simulink model "BLDC_120degree_speed_control"  (R2022b)
settings: Solver=VariableStepAuto  StartTime=0.0  StopTime=0.5  FixedStep=0.000001  MinStep=0.000001  RelTol=1e-3
values from neighbouring files (symbols this model uses):
  B = 0.0005    [bldc_params.m]
  J = 0.0002    [bldc_params.m]
  Lamda_p = Kb * pole/2    (= 0.1046)    [bldc_params.m]
  Ls_Lm = 5.21e-3    (= 0.00521)    [bldc_params.m]
  pole = 4    [bldc_params.m]
  Rs = 0.7    [bldc_params.m]
  T_rate = 1.78    [bldc_params.m]
libraries: slpidlib x1, spsTriangleGeneratorLib x1
settings Model: Creator=jack  LastModifiedBy=jack

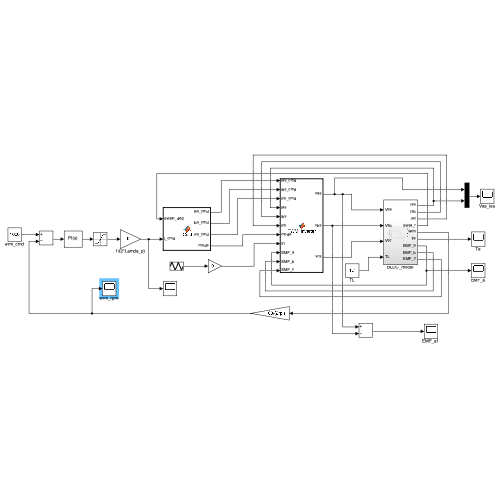
[thumbnail: Simulink's stored preview of the top-level diagram]
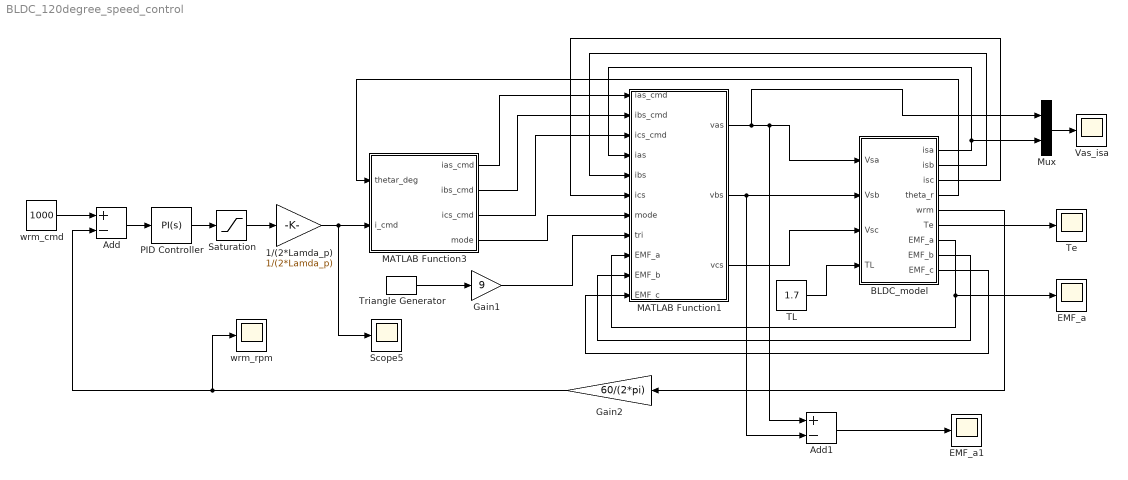
== system BLDC_120degree_speed_control ==
  1/(2*Lamda_p) : Gain  Gain=1/(2*Lamda_p)
  Add : Sum  Inputs=+-
  Add1 : Sum  Inputs=+-
  BLDC_model : Subsystem
  EMF_a : Scope
  EMF_a1 : Scope
  Gain1 : Gain  Gain=9
  Gain2 : Gain  Gain=60/(2*pi)
  MATLAB Function1 : MATLAB Function  TreatAsAtomicUnit=on
  MATLAB Function3 : MATLAB Function  TreatAsAtomicUnit=on
  Mux : Mux  Inputs=2
  PID Controller : slpidlib/PID Controller  Controller=PI  Form=Parallel  TimeDomain=Continuous-time  UseExternalTs=off  SampleTime=-1  IntegratorMethod=Forward Euler  FilterMethod=Forward Euler  ControllerParametersSource=internal  P=0.03  I=0.25  UseKiTs=off  D=0  N=100  UseFilter=on  TunerSelectOption=Transfer Function Based (PID Tuner App)  InitialConditionSource=internal  InitialConditionForIntegrator=0  InitialConditionForFilter=0  DifferentiatorICPrevScaledInput=0  ExternalReset=none  TrackingMode=off  Kt=1  LimitOutput=off  SatLimitsSource=internal  UpperSaturationLimit=inf  LowerSaturationLimit=-inf  LinearizeAsGain=on  AntiWindupMode=none  Kb=1  LimitIntegrator=off  UpperIntegratorSaturationLimit=inf  LowerIntegratorSaturationLimit=-inf  POutMin=[]  POutMax=[]  IOutMin=[]  IOutMax=[]  DOutMin=[]  DOutMax=[]  NOutMin=[]  NOutMax=[]  SumOutMin=[]  SumOutMax=[]  SaturationOutMin=[]  SaturationOutMax=[]  PParamMin=[]  PParamMax=[]  IParamMin=[]  IParamMax=[]  DParamMin=[]  DParamMax=[]  NParamMin=[]  NParamMax=[]  KbParamMin=[]  KbParamMax=[]  KtParamMin=[]  KtParamMax=[]  KbOutMin=[]  KbOutMax=[]  KtOutMin=[]  KtOutMax=[]  IntegratorOutMin=[]  IntegratorOutMax=[]  FilterOutMin=[]  FilterOutMax=[]  SumI1OutMin=[]  SumI1OutMax=[]  SumI2OutMin=[]  SumI2OutMax=[]  SumI3OutMin=[]  SumI3OutMax=[]  SumI4OutMin=[]  SumI4OutMax=[]  SumDOutMin=[]  SumDOutMax=[]  DifferentiatorOutMin=[]  DifferentiatorOutMax=[]  FilterDiffOutCoefMin=[]  FilterDiffOutCoefMax=[]  ReciprocalOutMin=[]  ReciprocalOutMax=[]  SumDenOutMin=[]  SumDenOutMax=[]  SumNumOutMin=[]  SumNumOutMax=[]  DivideOutMin=[]  DivideOutMax=[]  UdiffTsProdOutMin=[]  UdiffTsProdOutMax=[]  NTsProdOutMin=[]  NTsProdOutMax=[]  UintegralTsProdOutMin=[]  UintegralTsProdOutMax=[]  UngainTsProdOutMin=[]  UngainTsProdOutMax=[]  ClampingZeroOutDataTypeStr=Inherit: Inherit via back propagation  ClampingZeroOutMin=[]  ClampingZeroOutMax=[]  FilterDenConstantOutDataTypeStr=Inherit: Inherit via back propagation  FilterDenConstantOutMin=[]  FilterDenConstantOutMax=[]  PCopyOutDataTypeStr=Inherit: Inherit via back propagation  PCopyOutMin=[]  PCopyOutMax=[]  NCopyOutDataTypeStr=Inherit: Inherit via back propagation  NCopyOutMin=[]  NCopyOutMax=[]  IntegratorContinuousStateAttributes=''  IntegratorStateMustResolveToSignalObject=off  IntegratorRTWStateStorageClass=Auto  FilterContinuousStateAttributes=''  FilterStateMustResolveToSignalObject=off  FilterRTWStateStorageClass=Auto  ParallelPVariant=InternalParameters  IdealPVariant=Disabled  IVariant=InternalParameters  DVariant=Disabled  IntegratorVariant=Continuous  SatVariant=Disabled  AWVariant=Passthrough  PCopyVariant=Disabled  TRVariant=Disabled  FdbkBlocksVariant=Forward  IdealPFdbkVariant=Disabled  SatFdbkVariant=Disabled  DerivativeFilterVariant=Disabled  NVariant=Disabled  NCopyVariant=Disabled_SignalSpec  FilterICVariant=Disabled  IntegratorICVariant=InternalICs  ExternalResetVariant=Disabled  TRSumVariant=Passthrough  SumFdbkVariant=Disabled  SumVariant=Sum_PI  TsampFilterVariant=InternalTs  TsampNgainVariant=Passthrough  TsampIntegralVariant=Passthrough  ExternalSaturationOutDataTypeStr=Inherit: Same as second input
  Saturation : Saturate  UpperLimit=2*T_rate  LowerLimit=-2*T_rate
  Scope5 : Scope
  TL : Constant  Value=1.7
  Te : Scope
  Triangle Generator : spsTriangleGeneratorLib/Triangle Generator  Freq=4000  Phase=90  Ts=0
  Vas_isa : Scope
  wrm_cmd : Constant  Value=1000
  wrm_rpm : Scope
  wires:
  wrm_cmd/1 -> Add/1
  Add/1 -> PID Controller/1
  PID Controller/1 -> Saturation/1
  BLDC_model/5(wrm) -> Gain2/1
  1/(2*Lamda_p)/1 -> MATLAB Function3/2(i_cmd), Scope5/1
  MATLAB Function3/1(ias_cmd) -> MATLAB Function1/1(ias_cmd)
  MATLAB Function3/2(ibs_cmd) -> MATLAB Function1/2(ibs_cmd)
  MATLAB Function3/3(ics_cmd) -> MATLAB Function1/3(ics_cmd)
  MATLAB Function3/4(mode) -> MATLAB Function1/7(mode)
  BLDC_model/2(isb) -> MATLAB Function1/5(ibs)
  BLDC_model/3(isc) -> MATLAB Function1/6(ics)
  Triangle Generator/1 -> Gain1/1
  Gain1/1 -> MATLAB Function1/8(tri)
  MATLAB Function1/1(vas) -> Mux/1, Add1/1, BLDC_model/1(Vsa)
  MATLAB Function1/2(vbs) -> Add1/2, BLDC_model/2(Vsb)
  MATLAB Function1/3(vcs) -> BLDC_model/3(Vsc)
  TL/1 -> BLDC_model/4(TL)
  BLDC_model/4(theta_r) -> MATLAB Function3/1(thetar_deg)
  Gain2/1 -> wrm_rpm/1, Add/2
  BLDC_model/1(isa) -> MATLAB Function1/4(ias), Mux/2
  Saturation/1 -> 1/(2*Lamda_p)/1
  BLDC_model/9(EMF_c) -> MATLAB Function1/11(EMF_c)
  BLDC_model/8(EMF_b) -> MATLAB Function1/10(EMF_b)
  BLDC_model/7(EMF_a) -> EMF_a/1, MATLAB Function1/9(EMF_a)
  Mux/1 -> Vas_isa/1
  Add1/1 -> EMF_a1/1
  BLDC_model/6(Te) -> Te/1

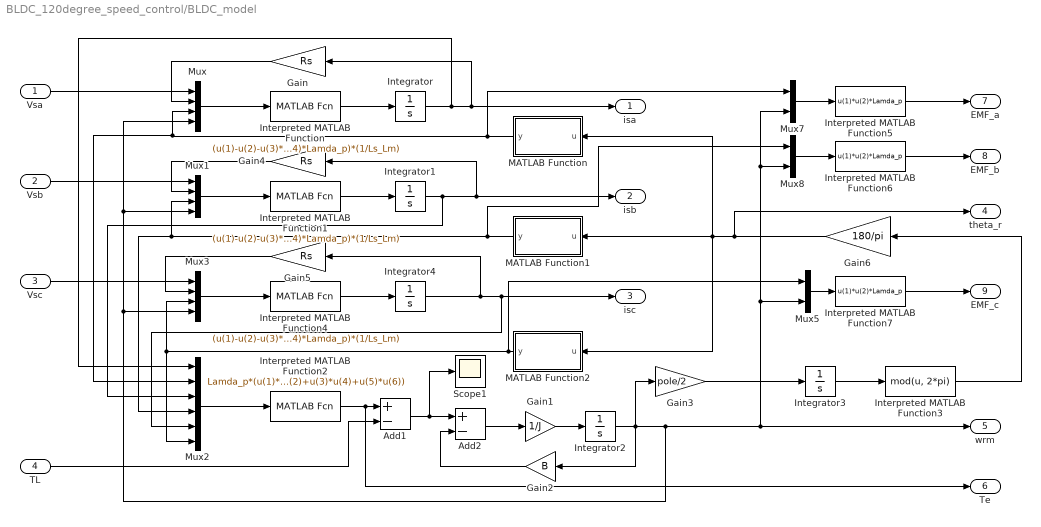
== system BLDC_120degree_speed_control/BLDC_model ==
  Vsa : Inport
  Vsb : Inport  Port=2
  Vsc : Inport  Port=3
  TL : Inport  Port=4
  Add1 : Sum  Inputs=+-
  Add2 : Sum  Inputs=+-
  Gain : Gain  Gain=Rs
  Gain1 : Gain  Gain=1/J
  Gain2 : Gain  Gain=B
  Gain3 : Gain  Gain=pole/2
  Gain4 : Gain  Gain=Rs
  Gain5 : Gain  Gain=Rs
  Gain6 : Gain  Gain=180/pi
  Integrator{,1..4} (5 alike) : Integrator
  Interpreted MATLAB Function : MATLABFcn  MATLABFcn=(u(1)-u(2)-u(3)*u(4)*Lamda_p)*(1/Ls_Lm)
  Interpreted MATLAB Function1 : MATLABFcn  MATLABFcn=(u(1)-u(2)-u(3)*u(4)*Lamda_p)*(1/Ls_Lm)
  Interpreted MATLAB Function2 : MATLABFcn  MATLABFcn=Lamda_p*(u(1)*u(2)+u(3)*u(4)+u(5)*u(6))
  Interpreted MATLAB Function3 : MATLABFcn  MATLABFcn=mod(u, 2*pi)
  Interpreted MATLAB Function4 : MATLABFcn  MATLABFcn=(u(1)-u(2)-u(3)*u(4)*Lamda_p)*(1/Ls_Lm)
  Interpreted MATLAB Function5 : MATLABFcn  MATLABFcn=u(1)*u(2)*Lamda_p
  Interpreted MATLAB Function6 : MATLABFcn  MATLABFcn=u(1)*u(2)*Lamda_p
  Interpreted MATLAB Function7 : MATLABFcn  MATLABFcn=u(1)*u(2)*Lamda_p
  MATLAB Function : MATLAB Function  TreatAsAtomicUnit=on
  MATLAB Function1 : MATLAB Function  TreatAsAtomicUnit=on
  MATLAB Function2 : MATLAB Function  TreatAsAtomicUnit=on
  Mux : Mux
  Mux1 : Mux
  Mux2 : Mux  Inputs=6
  Mux3 : Mux
  Mux5 : Mux  Inputs=2
  Mux7 : Mux  Inputs=2
  Mux8 : Mux  Inputs=2
  Scope1 : Scope
  isa : Outport
  isb : Outport  Port=2
  isc : Outport  Port=3
  theta_r : Outport  Port=4
  wrm : Outport  Port=5
  Te : Outport  Port=6
  EMF_a : Outport  Port=7
  EMF_b : Outport  Port=8
  EMF_c : Outport  Port=9
  wires:
  Gain5/1 -> Mux3/2
  Gain2/1 -> Add2/2
  Mux1/1 -> Interpreted MATLAB Function1/1
  Integrator2/1 -> Gain3/1, Mux1/4, Mux/4, Mux3/4, wrm/1, Mux7/2, Mux8/2, Mux5/2, Gain2/1
  Interpreted MATLAB Function/1 -> Integrator/1
  Add2/1 -> Gain1/1
  Integrator4/1 -> Gain5/1, isc/1, Mux2/5
  Vsa/1 -> Mux/1
  Gain1/1 -> Integrator2/1
  TL/1 -> Add1/2
  Vsc/1 -> Mux3/1
  Mux/1 -> Interpreted MATLAB Function/1
  Integrator3/1 -> Interpreted MATLAB Function3/1
  Gain4/1 -> Mux1/2
  Integrator1/1 -> Mux2/3, isb/1, Gain4/1
  Interpreted MATLAB Function4/1 -> Integrator4/1
  Interpreted MATLAB Function3/1 -> Gain6/1
  Add1/1 -> Scope1/1, Add2/1
  Interpreted MATLAB Function2/1 -> Te/1, Add1/1
  Mux3/1 -> Interpreted MATLAB Function4/1
  Interpreted MATLAB Function1/1 -> Integrator1/1
  Mux2/1 -> Interpreted MATLAB Function2/1
  MATLAB Function/1(y) -> Mux7/1, Mux2/2, Mux/3
  MATLAB Function1/1(y) -> Mux8/1, Mux1/3, Mux2/4
  Integrator/1 -> isa/1, Gain/1, Mux2/1
  Gain3/1 -> Integrator3/1
  MATLAB Function2/1(y) -> Mux2/6, Mux3/3, Mux5/1
  Gain/1 -> Mux/2
  Vsb/1 -> Mux1/1
  Gain6/1 -> theta_r/1, MATLAB Function/1(u), MATLAB Function2/1(u), MATLAB Function1/1(u)
  Mux7/1 -> Interpreted MATLAB Function5/1
  Interpreted MATLAB Function5/1 -> EMF_a/1
  Mux8/1 -> Interpreted MATLAB Function6/1
  Interpreted MATLAB Function6/1 -> EMF_b/1
  Mux5/1 -> Interpreted MATLAB Function7/1
  Interpreted MATLAB Function7/1 -> EMF_c/1

== matlab function BLDC_120degree_speed_control/BLDC_model/MATLAB Function1 ==
  data: u input; y output
function y = fbs(u)
    if ((u>=0) && (u<90))
        y = -1;
    elseif ((u>=90) && (u<150))
        y = u/30 - 4;
    elseif ((u>=150) && (u<270))
        y = 1;
    elseif ((u>=270) && (u<330))
        y = -u/30 + 10;
    elseif ((u>=330) && (u<=360))
        y = -1;
    else
        y = 0;
    end

== matlab function BLDC_120degree_speed_control/BLDC_model/MATLAB Function ==
  data: u input; y output
function y = fas(u)
    if ((u>=0) && (u<30))
        y = u/30;
    elseif ((u>=30) && (u<150))
        y = 1;
    elseif ((u>=150) && (u<210))
        y = -u/30 + 6;
    elseif ((u>=210) && (u<330))
        y = -1;
    elseif ((u>=330) && (u<=360))
        y = u/30 - 12;
    else 
        y = 0;
    end

== matlab function BLDC_120degree_speed_control/BLDC_model/MATLAB Function2 ==
  data: u input; y output
function y = fcs(u)
    if ((u>=0) && (u<30))
        y = 1;
    elseif ((u>=30) && (u<90))
        y = -u/30 + 2;
    elseif ((u>=90) && (u<210))
        y = -1;
    elseif ((u>=210) && (u<270))
        y = u/30 - 8;
    elseif ((u>=270) && (u<=360))
        y = 1;
    else
        y = 0;
    end

== matlab function BLDC_120degree_speed_control/MATLAB Function1 ==
  data: ias_cmd input; vas output; ibs_cmd input; ics_cmd input; ias input; ibs input; ics input; mode input; tri input; vbs output; vcs output; EMF_a input; EMF_b input; EMF_c input
function [vas, vbs, vcs] = PWM_inverter(ias_cmd, ibs_cmd, ics_cmd, ias, ibs, ics, mode, tri, EMF_a, EMF_b, EMF_c)
    kp_i = 100; vc_lim_p = 9; vc_lim_n = -9;
    vdc = 160; vas = 0; vbs = 0; vcs = 0;
    if ((mode~=1)&&(mode~=4))
        vasc = kp_i*(ias_cmd-ias);
        if (vasc > vc_lim_p)
            vasc = vc_lim_p;
        elseif (vasc < vc_lim_n)
            vasc = vc_lim_n;
        end
        if (vasc >= tri)
            vas = vdc/2;
        else
            vas = -vdc/2;
        end
    elseif (mode==4)
        if (ias > 0)
            vas = -vdc/2;
        else
            vas = EMF_a;
        end
    elseif (mode==1)
        if (ias<0)
            vas = vdc/2;
        else
            vas = EMF_a;
        end
    else
        vas = 0;
    end
    % for B phase control
    if ((mode~=3)&&(mode~=6))
        vbsc = kp_i*(ibs_cmd-ibs);
        if (vbsc > vc_lim_p)
            vbsc = vc_lim_p;
        elseif (vbsc < vc_lim_n)
            vbsc = vc_lim_n;
        end
        if (vbsc >= tri)
            vbs = vdc/2;
        else
            vbs = -vdc/2;
        end
    elseif (mode==6)
        if (ibs>0)
            vbs = -vdc/2;
        else
            vbs = EMF_b;
        end
    elseif (mode==3)
        if (ibs<0)
            vbs = vdc/2;
        else
            vbs = EMF_b;
        end
    else
        vbs = 0;
    end    
    % for C phase control
    if ((mode~=5)&&(mode~=2))
        vcsc = kp_i*(ics_cmd-ics);
        if (vcsc > vc_lim_p)
            vcsc = vc_lim_p;
        elseif (vcsc < vc_lim_n)
            vcsc = vc_lim_n;
        end
        if (vcsc >= tri)
            vcs = vdc/2;
        else
            vcs = -vdc/2;
        end
    elseif (mode==2)
        if (ics>0)
            vcs = -vdc/2;
        else
            vcs = EMF_c;
        end
    elseif (mode==5)
        if (ics<0)
            vcs = vdc/2;
        else
            vcs = EMF_c;
        end
    else
        vcs = 0;
    end

== matlab function BLDC_120degree_speed_control/MATLAB Function3 ==
  data: thetar_deg input; ias_cmd output; i_cmd input; ibs_cmd output; ics_cmd output; mode output
function [ias_cmd, ibs_cmd, ics_cmd, mode] = iCmd(thetar_deg, i_cmd)
    if (((thetar_deg>=0) && (thetar_deg<30))||((thetar_deg>=330) && (thetar_deg<=360)))
        mode = 1;
        ias_cmd = 0;
        ibs_cmd = -i_cmd;
        ics_cmd = i_cmd;
    elseif ((thetar_deg>=30) && (thetar_deg<90))
        mode = 2;
        ias_cmd = i_cmd;
        ibs_cmd = -i_cmd;
        ics_cmd = 0;
    elseif ((thetar_deg>=90) && (thetar_deg<150))
        mode = 3;
        ias_cmd = i_cmd;
        ibs_cmd = 0;
        ics_cmd = -i_cmd;  
    elseif ((thetar_deg>=150) && (thetar_deg<210))
        mode = 4;
        ias_cmd = 0;
        ibs_cmd = i_cmd;
        ics_cmd = -i_cmd;          
    elseif ((thetar_deg>=210) && (thetar_deg<270))
        mode = 5;
        ias_cmd = -i_cmd;
        ibs_cmd = i_cmd;
        ics_cmd = 0;  
    elseif ((thetar_deg>=270) && (thetar_deg<330))
        mode = 6;
        ias_cmd = -i_cmd;
        ibs_cmd = 0;
        ics_cmd = i_cmd;  
    else
        mode = 0;
        ias_cmd = 0;
        ibs_cmd = 0;
        ics_cmd = 0;          
    end
